simulink model "angle_estimision"  (R2021a)
settings: Solver=VariableStepAuto  StartTime=0.0  StopTime=330  RelTol=1e-3
values from neighbouring files (symbols this model uses):
  IMU_params =     [IMU_params.mat]
settings Model: Creator=Administrator  LastModifiedBy=Administrator

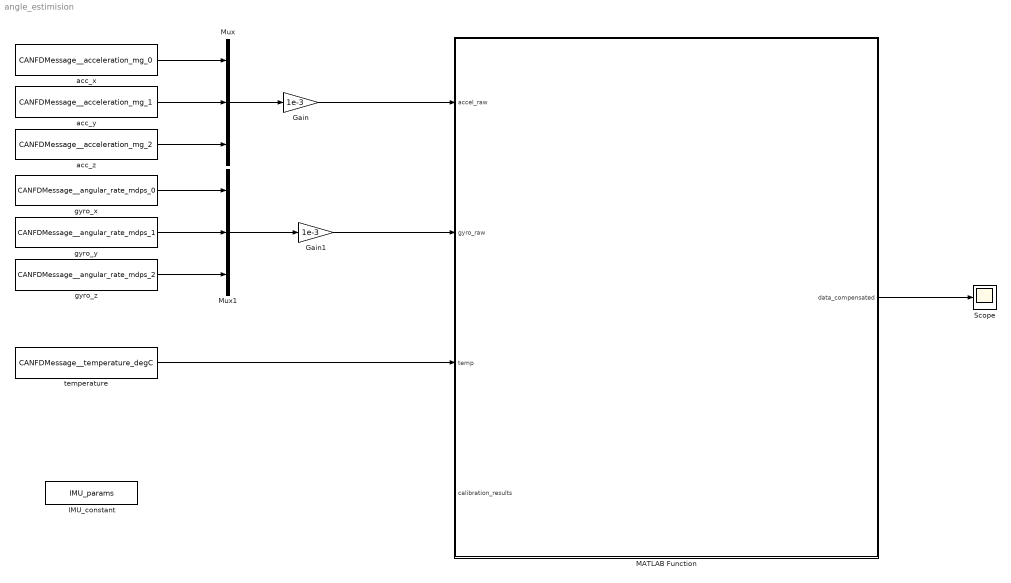
== system angle_estimision ==
  Gain : Gain  Gain=1e-3
  Gain1 : Gain  Gain=1e-3
  IMU_constant : Constant  Value=IMU_params  VectorParams1D=off
  MATLAB Function : MATLAB Function  TreatAsAtomicUnit=on
  Mux : Mux  Inputs=3
  Mux1 : Mux  Inputs=3
  Scope : Scope
  acc_x : FromWorkspace  VariableName=CANFDMessage__acceleration_mg_0  SampleTime=-1
  acc_y : FromWorkspace  VariableName=CANFDMessage__acceleration_mg_1  SampleTime=-1
  acc_z : FromWorkspace  VariableName=CANFDMessage__acceleration_mg_2  SampleTime=-1
  gyro_x : FromWorkspace  VariableName=CANFDMessage__angular_rate_mdps_0  SampleTime=-1
  gyro_y : FromWorkspace  VariableName=CANFDMessage__angular_rate_mdps_1  SampleTime=-1
  gyro_z : FromWorkspace  VariableName=CANFDMessage__angular_rate_mdps_2  SampleTime=-1
  temperature : FromWorkspace  VariableName=CANFDMessage__temperature_degC  SampleTime=-1
  wires:
  acc_x/1 -> Mux/1
  acc_y/1 -> Mux/2
  acc_z/1 -> Mux/3
  Mux/1 -> Gain/1
  gyro_z/1 -> Mux1/3
  gyro_y/1 -> Mux1/2
  gyro_x/1 -> Mux1/1
  Mux1/1 -> Gain1/1
  temperature/1 -> MATLAB Function/3(temp)
  Gain/1 -> MATLAB Function/1(accel_raw)
  Gain1/1 -> MATLAB Function/2(gyro_raw)
  MATLAB Function/1(data_compensated) -> Scope/1

== matlab function angle_estimision/MATLAB Function ==
  data: accel_raw input; data_compensated output; gyro_raw input; temp input; calibration_results input
function data_compensated  = imu_preprocessing(accel_raw, gyro_raw, temp, calibration_results)
% IMU信号预处理函数：实现滤波与误差补偿
% 输入：
%   accel_raw       - 原始加速度计数据 [3×1] (m/s²)
%   gyro_raw        - 原始陀螺仪数据 [3×1] (rad/s)
%   temp            - 当前IMU温度 (℃)
%   dt              - 采样时间间隔 (s)
%   accel_params    - 加速度计误差参数结构体，包含：
%       .bias        - 零偏 [3×1] (m/s²)
%       .temp_coeff  - 温度系数 [3×1] (m/s²/℃)
%       .scale_mat   - 刻度矩阵 [3×3]
%       .filter_alpha- 低通滤波系数 (0~1，推荐0.2~0.5)
%   gyro_params     - 陀螺仪误差参数结构体，包含：
%       .bias        - 零偏 [3×1] (rad/s)
%       .temp_coeff  - 温度系数 [3×1] (rad/s/℃)
%       .scale_mat   - 刻度矩阵 [3×3]
%       .filter_alpha- 低通滤波系数 (0~1，推荐0.1~0.3)
% 输出：
%   accel_compensated - 补偿后加速度 [3×1] (m/s²)
%   gyro_compensated  - 补偿后角速度 [3×1] (rad/s)

accel_filter_alpha = 0.3;  % 加速度计滤波系数（固定值）
gyro_filter_alpha = 0.2;   % 陀螺仪滤波系数（固定值）
% 持久化变量：存储滤波历史值（Simulink中保持状态）
persistent accel_filtered_prev gyro_filtered_prev
if isempty(accel_filtered_prev)
    accel_filtered_prev = zeros(3,1);  % 加速度滤波历史值
end
if isempty(gyro_filtered_prev)
    gyro_filtered_prev = zeros(3,1);   % 角速度滤波历史值
end

%% 1. 信号滤波（一阶低通滤波，抑制高频噪声）
% 加速度计滤波：y(k) = α*y(k-1) + (1-α)*x(k)
accel_filtered = accel_filter_alpha * accel_filtered_prev + ...
                 (1 - accel_params.filter_alpha) * accel_raw;
% 陀螺仪滤波
gyro_filtered = gyro_filter_alpha * gyro_filtered_prev + ...
                (1 - gyro_params.filter_alpha) * gyro_raw;

%% 2. 误差补偿（零偏+温度+刻度误差）
% 温度偏差（基准温度25℃，与标定一致）
% delta_T = temp - 25;

% 2.1 加速度计补偿
accel_no_bias_temp = accel_filtered - calibration_results.accel.bias;
accel_compensated = pinv(calibration_results.accel.scale_mat) * accel_no_bias_temp;
% 2.2 陀螺仪补偿
gyro_no_bias_temp = gyro_filtered - calibration_results.gyro.bias;
gyro_compensated = pinv(calibration_results.gyro.scale_mat) * gyro_no_bias_temp;


data_compensated = [accel_compensated; gyro_compensated];

%% 更新历史值（用于下一时刻滤波）
accel_filtered_prev = accel_filtered;
gyro_filtered_prev = gyro_filtered;

end
